simulink model "week2_prob3"  (R2021a)
settings: Solver=VariableStepAuto  StartTime=0.0  StopTime=50  RelTol=1e-3
settings Model: DataDictionary=week2_prob3.sldd  Creator=varunraj  LastModifiedBy=varunraj

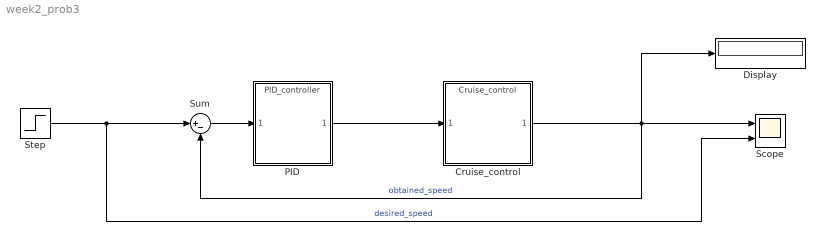
== system week2_prob3 ==
  Cruise_control : ModelReference  ModelNameDialog=Cruise_control  SimulationMode=Normal  ModelReferenceVersion=1.2
  Display : Display
  PID : ModelReference  ModelNameDialog=PID_controller  SimulationMode=Normal  ModelReferenceVersion=1.2
  Scope : Scope  NumInputPorts=2
  Step : Step  After=u  SampleTime=0
  Sum : Sum  Inputs=|+-
  wires:
  Sum/1 -> PID/1
  Step/1 -> Scope/2, Sum/1  "desired_speed"
  PID/1 -> Cruise_control/1
  Cruise_control/1 -> Sum/2, Display/1, Scope/1  "obtained_speed"
